simulink model "bloodver1"  (R2022a)
settings: Solver=VariableStepAuto  StartTime=0.0  StopTime=10.0  RelTol=1e-3
libraries: simulink x8
settings Model: Creator=theva  LastModifiedBy=theva

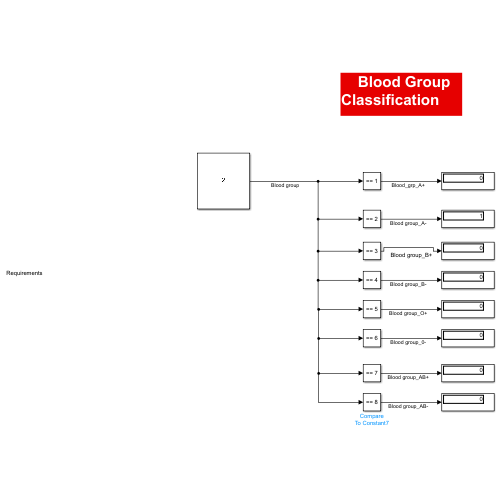
[thumbnail: Simulink's stored preview of the top-level diagram]
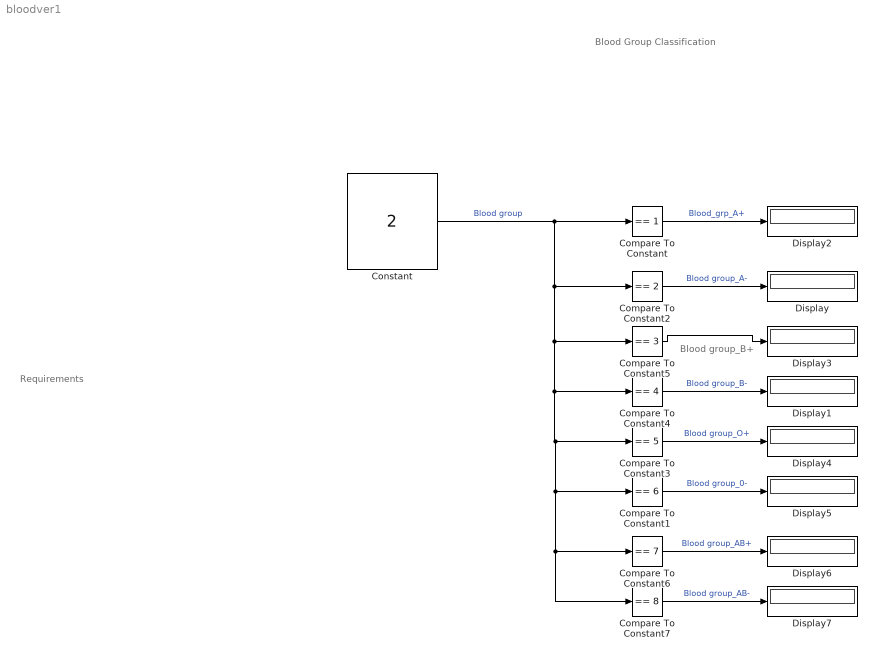
== system bloodver1 ==
  note: Requirements
  note: Blood group_B+
  note: Blood Group Classification
  Compare To Constant : simulink/Logic and Bit Operations/Compare To Constant  relop===  const=1  OutDataTypeStr=boolean
  Compare To Constant1 : simulink/Logic and Bit Operations/Compare To Constant  relop===  const=6  OutDataTypeStr=boolean
  Compare To Constant2 : simulink/Logic and Bit Operations/Compare To Constant  relop===  const=2  OutDataTypeStr=boolean
  Compare To Constant3 : simulink/Logic and Bit Operations/Compare To Constant  relop===  const=5  OutDataTypeStr=boolean
  Compare To Constant4 : simulink/Logic and Bit Operations/Compare To Constant  relop===  const=4  OutDataTypeStr=boolean
  Compare To Constant5 : simulink/Logic and Bit Operations/Compare To Constant  relop===  const=3  OutDataTypeStr=boolean
  Compare To Constant6 : simulink/Logic and Bit Operations/Compare To Constant  relop===  const=7  OutDataTypeStr=boolean
  Compare To Constant7 : simulink/Logic and Bit Operations/Compare To Constant  relop===  const=8  OutDataTypeStr=boolean
  Constant : Constant  Value=2
  Display{,1..7} (8 alike) : Display
  wires:
  Constant/1 -> Compare To Constant7/1, Compare To Constant6/1, Compare To Constant1/1, Compare To Constant3/1, Compare To Constant4/1, Compare To Constant5/1, Compare To Constant2/1, Compare To Constant/1  "Blood group"
  Compare To Constant/1 -> Display2/1  "Blood_grp_A+"
  Compare To Constant2/1 -> Display/1  "Blood group_A-"
  Compare To Constant5/1 -> Display3/1
  Compare To Constant4/1 -> Display1/1  "Blood group_B-"
  Compare To Constant3/1 -> Display4/1  "Blood group_O+"
  Compare To Constant1/1 -> Display5/1  "Blood group_0-"
  Compare To Constant6/1 -> Display6/1  "Blood group_AB+"
  Compare To Constant7/1 -> Display7/1  "Blood group_AB-"
